simulink model "surge_model"  (R2014a)
settings: Solver=ode45  StartTime=tstart  StopTime=tstop  RelTol=1e-3
values from neighbouring files (symbols this model uses):
  nc = 80*2*pi/60    (= 8.37758040957)    [run_task_1_6.m]
undefined symbols (not defined in the file or in its folder): T
settings Model: Creator=Hwk  LastModifiedBy=Hwk

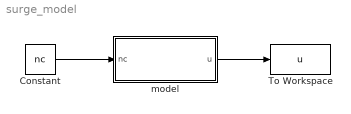
== system surge_model ==
  Constant : Constant  Value=nc
  To Workspace : ToWorkspace  VariableName=u  SampleTime=10
  model : Subsystem
  wires:
  model/1(u) -> To Workspace/1
  Constant/1 -> model/1(nc)

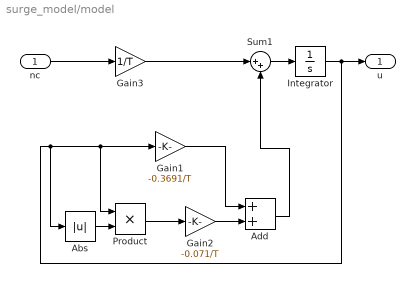
== system surge_model/model ==
  nc : Inport
  Abs : Abs
  Add : Sum
  Gain1 : Gain  Gain=-0.3691/T
  Gain2 : Gain  Gain=-0.071/T
  Gain3 : Gain  Gain=1/T
  Integrator : Integrator
  Product : Product
  Sum1 : Sum  Inputs=|++
  u : Outport
  wires:
  nc/1 -> Gain3/1
  Gain3/1 -> Sum1/1
  Gain1/1 -> Add/1
  Sum1/1 -> Integrator/1
  Product/1 -> Gain2/1
  Gain2/1 -> Add/2
  Add/1 -> Sum1/2
  Integrator/1 -> Gain1/1, Product/1, Abs/1, u/1
  Abs/1 -> Product/2
